simulink subsystem "RRR_rigid_joints_"  (R2021b)
settings: Solver=VariableStepAuto  StartTime=0.0  StopTime=10.0  RelTol=1e-3
undefined symbols (not defined in the file): q0, qd0
settings Model: Creator=fabioscap  LastModifiedBy=fabioscap

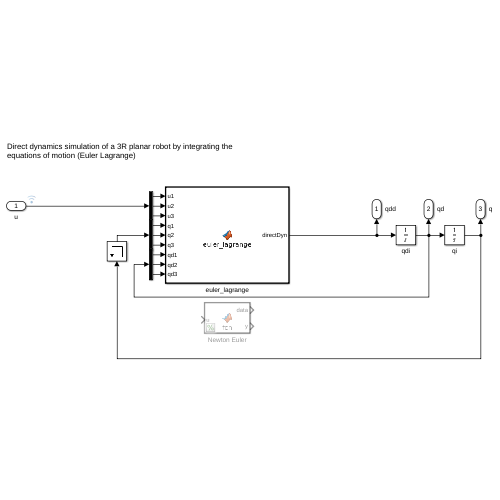
[thumbnail: Simulink's stored preview of the top-level diagram]
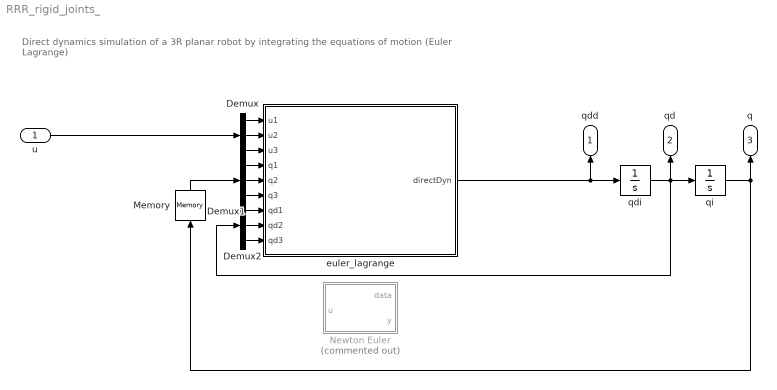
== system RRR_rigid_joints_ ==
  note: Direct dynamics simulation of a 3R planar robot by integrating the equations of motion (Euler Lagrange)
  u : Inport  PortDimensions=3
  Demux : Demux  Outputs=3
  Demux1 : Demux  Outputs=3
  Demux2 : Demux  Outputs=3
  Memory : Memory
  Newton Euler : MATLAB Function  Commented=on  TreatAsAtomicUnit=on
  euler_lagrange : MATLAB Function  TreatAsAtomicUnit=on
  qdi : Integrator  InitialCondition=qd0
  qi : Integrator  InitialCondition=q0
  qdd : Outport
  qd : Outport  Port=2
  q : Outport  Port=3  PortDimensions=3
  wires:
  Demux/2 -> euler_lagrange/2(u2)
  u/1 -> Demux/1
  Demux2/3 -> euler_lagrange/9(qd3)
  Demux/3 -> euler_lagrange/3(u3)
  euler_lagrange/1(directDyn) -> qdi/1, qdd/1
  Demux1/3 -> euler_lagrange/6(q3)
  Demux1/2 -> euler_lagrange/5(q2)
  qi/1 -> Memory/1, q/1
  Demux2/2 -> euler_lagrange/8(qd2)
  Memory/1 -> Demux1/1
  Demux2/1 -> euler_lagrange/7(qd1)
  qdi/1 -> Demux2/1, qi/1, qd/1
  Demux1/1 -> euler_lagrange/4(q1)
  Demux/1 -> euler_lagrange/1(u1)

== matlab function RRR_rigid_joints_/euler_lagrange ==
  data: u1 input; directDyn output; u2 input; u3 input; q1 input; q2 input; q3 input; qd1 input; qd2 input; qd3 input
function directDyn = euler_lagrange(u1,u2,u3,q1,q2,q3,qd1,qd2,qd3)
%#codegen

%    This function was generated by the Symbolic Math Toolbox version 9.0.
%    22-Jul-2022 17:48:26

t2 = cos(q2);
t3 = cos(q3);
t4 = sin(q2);
t5 = sin(q3);
t6 = q2+q3;
t7 = qd1.^2;
t8 = qd2.^2;
t9 = qd3.^2;
t16 = u1.*8.0;
t10 = t2.^2;
t11 = t3.^2;
t12 = t5.^2;
t13 = t5.^3;
t14 = cos(t6);
t15 = sin(t6);
t20 = t2.*u1.*1.2e+1;
t21 = t2.*u2.*1.2e+1;
t22 = t2.*u3.*1.2e+1;
t25 = qd1.*qd2.*t4.*2.4e+1;
t26 = qd1.*qd3.*t5.*3.2e+1;
t27 = qd2.*qd3.*t5.*3.2e+1;
t33 = t4.*t8.*1.2e+1;
t34 = t5.*t9.*1.6e+1;
t41 = t2.*t3.*u3.*1.8e+1;
t54 = t2.*t5.*t7.*6.0;
t55 = t2.*t5.*t8.*6.0;
t56 = t2.*t5.*t9.*6.0;
t60 = qd1.*qd2.*t2.*t5.*1.2e+1;
t61 = qd1.*qd3.*t2.*t5.*1.2e+1;
t62 = qd2.*qd3.*t2.*t5.*1.2e+1;
t63 = qd1.*qd2.*t2.*t4.*3.6e+1;
t73 = t2.*t4.*t7.*1.8e+1;
t74 = t2.*t4.*t8.*1.8e+1;
t91 = qd1.*qd2.*t2.*t3.*t5.*1.8e+1;
t110 = t2.*t3.*t5.*t7.*9.0;
t111 = t2.*t3.*t5.*t8.*9.0;
t17 = t14.^2;
t18 = t15.^2;
t19 = t15.^3;
t23 = t11.*u1.*6.0;
t24 = t11.*u2.*6.0;
t28 = t10.*9.0;
t29 = t11.*1.2e+1;
t30 = t12.*4.8e+1;
t31 = -t21;
t35 = t12.*u1.*2.4e+1;
t36 = t12.*u2.*2.4e+1;
t37 = -t26;
t38 = -t27;
t40 = t14.*u3.*1.2e+1;
t43 = -t34;
t45 = t3.*t14.*u1.*6.0;
t46 = t3.*t14.*u2.*6.0;
t47 = t3.*t14.*u3.*6.0;
t51 = t7.*t15.*4.0;
t52 = t8.*t15.*4.0;
t53 = t9.*t15.*4.0;
t57 = qd1.*qd2.*t15.*8.0;
t58 = qd1.*qd3.*t15.*8.0;
t59 = qd2.*qd3.*t15.*8.0;
t65 = t5.*t15.*u1.*2.4e+1;
t66 = t5.*t15.*u2.*2.4e+1;
t67 = t5.*t15.*u3.*2.4e+1;
t70 = -t54;
t71 = -t55;
t72 = -t56;
t75 = -t60;
t76 = -t61;
t77 = -t62;
t78 = qd1.*qd2.*t4.*t11.*1.8e+1;
t80 = t2.*t3.*t14.*9.0;
t81 = t2.*t7.*t15.*6.0;
t82 = t5.*t7.*t14.*6.0;
t83 = t2.*t8.*t15.*6.0;
t84 = t5.*t8.*t14.*6.0;
t85 = t2.*t9.*t15.*6.0;
t86 = qd1.*qd2.*t2.*t15.*1.2e+1;
t87 = qd1.*qd2.*t5.*t14.*1.2e+1;
t88 = qd1.*qd3.*t2.*t15.*1.2e+1;
t89 = qd2.*qd3.*t2.*t15.*1.2e+1;
t90 = t2.*t5.*t15.*3.6e+1;
t93 = qd1.*qd2.*t11.*t15.*6.0;
t94 = qd1.*qd3.*t11.*t15.*6.0;
t96 = qd2.*qd3.*t11.*t15.*6.0;
t98 = t3.*t5.*t15.*u3.*3.6e+1;
t99 = t4.*t7.*t11.*9.0;
t100 = t4.*t8.*t11.*9.0;
t101 = t4.*t7.*t12.*3.6e+1;
t102 = t4.*t8.*t12.*3.6e+1;
t103 = qd1.*qd2.*t4.*t12.*7.2e+1;
t104 = qd1.*qd2.*t3.*t5.*t14.*6.0;
t105 = qd1.*qd3.*t3.*t5.*t14.*6.0;
t106 = qd2.*qd3.*t3.*t5.*t14.*6.0;
t108 = t3.*t7.*t15.*2.4e+1;
t109 = t12.*t14.*u3.*3.6e+1;
t113 = -t91;
t114 = t7.*t11.*t15.*3.0;
t115 = t8.*t11.*t15.*3.0;
t116 = t9.*t11.*t15.*3.0;
t120 = qd1.*qd2.*t13.*t14.*3.6e+1;
t121 = t7.*t14.*t15.*6.0;
t122 = t3.*t5.*t7.*t14.*3.0;
t123 = t3.*t5.*t8.*t14.*3.0;
t124 = t3.*t5.*t9.*t14.*3.0;
t128 = qd1.*qd2.*t3.*t4.*t14.*1.8e+1;
t133 = -t110;
t134 = -t111;
t137 = t7.*t13.*t14.*1.8e+1;
t139 = t8.*t13.*t14.*1.8e+1;
t141 = qd1.*qd2.*t3.*t14.*t15.*6.0;
t142 = qd1.*qd3.*t3.*t14.*t15.*6.0;
t143 = qd2.*qd3.*t3.*t14.*t15.*6.0;
t147 = t3.*t4.*t7.*t14.*9.0;
t148 = t2.*t3.*t7.*t15.*9.0;
t149 = t3.*t4.*t8.*t14.*9.0;
t150 = t4.*t5.*t7.*t15.*3.6e+1;
t151 = t4.*t5.*t8.*t15.*3.6e+1;
t152 = qd1.*qd2.*t4.*t5.*t15.*7.2e+1;
t153 = qd1.*qd2.*t3.*t12.*t15.*3.6e+1;
t156 = t3.*t7.*t14.*t15.*3.0;
t157 = t3.*t8.*t14.*t15.*3.0;
t158 = t3.*t9.*t14.*t15.*3.0;
t159 = t3.*t5.*t14.*t15.*1.8e+1;
t163 = t2.*t7.*t14.*t15.*9.0;
t165 = t3.*t7.*t12.*t15.*1.8e+1;
t167 = t3.*t8.*t12.*t15.*1.8e+1;
t169 = qd1.*qd2.*t12.*t14.*t15.*3.6e+1;
t174 = t7.*t12.*t14.*t15.*1.8e+1;
t176 = t8.*t12.*t14.*t15.*1.8e+1;
t32 = -t24;
t39 = t17.*3.0;
t42 = -t28;
t44 = -t36;
t48 = t18.*1.2e+1;
t49 = -t40;
t50 = t17.*u2.*6.0;
t64 = -t46;
t69 = t18.*u2.*2.4e+1;
t79 = -t66;
t95 = qd1.*qd3.*t5.*t17.*6.0;
t97 = qd2.*qd3.*t5.*t17.*6.0;
t107 = -t80;
t112 = -t90;
t125 = -t104;
t126 = -t105;
t127 = -t106;
t129 = t12.*t17.*9.0;
t130 = t11.*t18.*9.0;
t131 = -t108;
t132 = -t109;
t135 = t5.*t9.*t17.*-3.0;
t136 = t4.*t7.*t17.*9.0;
t138 = t3.*t7.*t19.*1.8e+1;
t140 = t4.*t7.*t18.*3.6e+1;
t144 = -t122;
t145 = -t123;
t146 = -t124;
t154 = qd1.*qd2.*t3.*t5.*t18.*3.6e+1;
t160 = -t148;
t161 = -t153;
t164 = -t159;
t166 = t3.*t5.*t7.*t18.*1.8e+1;
t168 = t3.*t5.*t8.*t18.*1.8e+1;
t170 = -t165;
t172 = -t167;
t175 = t5.*t7.*t14.*t18.*1.8e+1;
t68 = -t50;
t92 = -t69;
t117 = t5.*t9.*t39;
t118 = -t95;
t119 = -t97;
t155 = -t138;
t162 = -t154;
t171 = -t166;
t173 = -t168;
t177 = t29+t30+t39+t42+t48+t107+t112+t129+t130+t164+1.6e+1;
t178 = 1.0./t177;
et1 = t16+t20+t22+t23+t25+t32+t33+t35+t37+t38+t41+t43+t44+t45+t47+t49+t51+t52+t53+t57+t58+t59+t63+t65+t67+t68+t70+t71+t72+t74+t75+t76+t77+t78+t81+t82+t83+t84+t85+t86+t87+t88+t89+t92+t93+t94+t96+t98+t99+t100+t101+t102+t103+t113+t114+t115+t116+t118+t119+t120+t121+t125+t126+t127+t128+t131+t132+t133+t134+t135+t136+t137+t139+t140+t141+t142+t143+t144+t145+t146+t149+t151+t152+t155+t156+t157+t158+t160+t161+t162+t163+t169+t170+t172+t173+t175+t176-u2.*4.0e+1+u3.*3.2e+1+t4.*t7.*6.0e+1-t5.*t7.*1.6e+1-t5.*t8.*1.6e+1-t2.*u2.*2.4e+1+t3.*u3.*4.8e+1+t17.*u3.*6.0+t18.*u3.*2.4e+1-qd1.*qd2.*t5.*3.2e+1+t2.*t4.*t7.*3.6e+1-t3.*t5.*t7.*2.4e+1-t3.*t5.*t8.*2.4e+1-t5.*t7.*t17.*3.0-t5.*t8.*t17.*3.0-t2.*t14.*u3.*1.8e+1-t3.*t14.*u2.*1.2e+1;
et2 = t5.*t15.*u2.*-4.8e+1+t3.*t18.*u3.*3.6e+1-qd1.*qd2.*t3.*t5.*4.8e+1-qd1.*qd2.*t5.*t17.*6.0+t2.*t5.*t7.*t14.*9.0+t3.*t4.*t7.*t14.*1.8e+1+t2.*t5.*t8.*t14.*9.0+t4.*t5.*t7.*t15.*7.2e+1-t3.*t5.*t7.*t18.*3.6e+1+t7.*t12.*t14.*t15.*3.6e+1-t5.*t14.*t15.*u3.*3.6e+1+qd1.*qd2.*t2.*t5.*t14.*1.8e+1;
et3 = t20+t31+t37+t38+t43+t45+t63+t64+t65+t68+t73+t74+t79+t81+t83+t85+t86+t88+t89+t92+t118+t119-t121+t128+t131+t135+t136+t140+t141+t142+t143+t147+t148+t149+t150+t151+t152+t155+t156+t157+t158+t162+t163+t169+t171+t173+t174+t175+t176-u2.*3.2e+1+u3.*6.4e+1+t4.*t7.*4.8e+1-t5.*t7.*3.2e+1-t5.*t8.*3.2e+1-t7.*t13.*4.8e+1-t8.*t13.*4.8e+1-t7.*t15.*1.6e+1-t7.*t19.*1.2e+1-t3.*u2.*4.8e+1+t3.*u3.*9.6e+1-t10.*u3.*1.8e+1+t11.*u3.*9.6e+1+t12.*u3.*9.6e+1-t14.*u1.*1.2e+1+t14.*u2.*1.2e+1+t17.*u3.*3.0e+1+t18.*u3.*4.8e+1-qd1.*qd2.*t5.*6.4e+1-qd1.*qd2.*t13.*9.6e+1+t3.*t4.*t7.*7.2e+1-t3.*t5.*t7.*4.8e+1-t3.*t5.*t8.*4.8e+1-t3.*t5.*t9.*2.4e+1;
et4 = t5.*t7.*t11.*-4.8e+1-t5.*t8.*t11.*4.8e+1-t4.*t7.*t14.*1.8e+1-t4.*t8.*t14.*1.8e+1-t5.*t7.*t17.*1.5e+1-t5.*t7.*t18.*1.2e+1-t5.*t8.*t17.*1.5e+1-t5.*t8.*t18.*1.2e+1-t7.*t11.*t15.*4.8e+1-t7.*t12.*t15.*4.8e+1-t7.*t11.*t19.*3.6e+1-t7.*t13.*t17.*3.6e+1-t8.*t14.*t15.*6.0-t8.*t13.*t17.*3.6e+1-t9.*t14.*t15.*6.0-t7.*t15.*t17.*1.2e+1+t5.*t7.*t28+t5.*t8.*t28+t7.*t15.*t28+t2.*t3.*u1.*1.8e+1-t2.*t3.*u2.*1.8e+1+t2.*t14.*u2.*1.8e+1-t2.*t14.*u3.*3.6e+1-t3.*t18.*u2.*3.6e+1+t3.*t18.*u3.*7.2e+1-t12.*t14.*u1.*3.6e+1+t12.*t14.*u2.*3.6e+1+t11.*t18.*u3.*7.2e+1+t12.*t17.*u3.*7.2e+1-qd1.*qd2.*t3.*t5.*9.6e+1;
et5 = qd1.*qd3.*t3.*t5.*-4.8e+1-qd2.*qd3.*t3.*t5.*4.8e+1+qd1.*qd2.*t5.*t10.*1.8e+1-qd1.*qd2.*t5.*t11.*9.6e+1-qd1.*qd2.*t4.*t14.*3.6e+1-qd1.*qd2.*t5.*t17.*3.0e+1-qd1.*qd2.*t5.*t18.*2.4e+1-qd1.*qd2.*t14.*t15.*1.2e+1-qd1.*qd2.*t13.*t17.*7.2e+1-qd1.*qd3.*t14.*t15.*1.2e+1-qd2.*qd3.*t14.*t15.*1.2e+1+t2.*t3.*t4.*t7.*2.7e+1+t2.*t3.*t4.*t8.*2.7e+1-t2.*t4.*t7.*t14.*2.7e+1+t2.*t3.*t8.*t15.*9.0+t2.*t5.*t7.*t14.*1.8e+1+t2.*t3.*t9.*t15.*9.0+t2.*t5.*t8.*t14.*1.8e+1+t2.*t5.*t9.*t14.*9.0+t2.*t5.*t7.*t18.*3.6e+1+t3.*t4.*t7.*t18.*5.4e+1+t2.*t7.*t12.*t15.*3.6e+1+t2.*t8.*t12.*t15.*3.6e+1-t4.*t7.*t12.*t14.*5.4e+1-t4.*t8.*t12.*t14.*5.4e+1-t5.*t7.*t11.*t18.*3.6e+1;
et6 = t5.*t8.*t11.*t18.*-3.6e+1-t7.*t12.*t15.*t17.*3.6e+1-t2.*t3.*t14.*u3.*7.2e+1+t3.*t5.*t15.*u1.*3.6e+1-t2.*t5.*t15.*u3.*7.2e+1-t3.*t5.*t15.*u2.*3.6e+1+t5.*t14.*t15.*u2.*3.6e+1-t5.*t14.*t15.*u3.*7.2e+1+qd1.*qd2.*t2.*t3.*t4.*5.4e+1+qd1.*qd2.*t2.*t3.*t15.*1.8e+1+qd1.*qd2.*t2.*t5.*t14.*3.6e+1+qd1.*qd3.*t2.*t3.*t15.*1.8e+1+qd1.*qd3.*t2.*t5.*t14.*1.8e+1+qd2.*qd3.*t2.*t3.*t15.*1.8e+1+qd2.*qd3.*t2.*t5.*t14.*1.8e+1+qd1.*qd2.*t2.*t12.*t15.*7.2e+1-qd1.*qd2.*t4.*t12.*t14.*1.08e+2-qd1.*qd2.*t5.*t11.*t18.*7.2e+1+t2.*t3.*t5.*t7.*t14.*3.6e+1+t2.*t3.*t5.*t8.*t14.*3.6e+1+t3.*t4.*t5.*t7.*t15.*5.4e+1+t3.*t4.*t5.*t8.*t15.*5.4e+1+t2.*t3.*t7.*t14.*t15.*3.6e+1-t4.*t5.*t7.*t14.*t15.*5.4e+1;
et7 = t3.*t5.*t7.*t14.*t18.*7.2e+1+t3.*t7.*t12.*t14.*t15.*7.2e+1+t3.*t8.*t12.*t14.*t15.*7.2e+1-t3.*t5.*t14.*t15.*u3.*1.44e+2+qd1.*qd2.*t2.*t3.*t5.*t14.*7.2e+1+qd1.*qd2.*t3.*t4.*t5.*t15.*1.08e+2+qd1.*qd2.*t3.*t12.*t14.*t15.*1.44e+2;
directDyn = [t178.*(t16+t22+t23+t25+t31+t32+t33+t35+t41+t44+t47+t49+t51+t52+t53+t57+t58+t59+t64+t67+t70+t71+t72+t73+t75+t76+t77+t78+t79+t82+t84+t87+t93+t94+t96+t98+t99+t100+t101+t102+t103+t113+t114+t115+t116+t120+t121+t125+t126+t127+t132+t133+t134+t137+t139+t144+t145+t146+t147+t150+t160+t161+t170+t171+t172+t174-u2.*8.0+t4.*t7.*1.2e+1).*(3.0./2.0);t178.*(et1+et2).*(-3.0./2.0);t178.*(et3+et4+et5+et6+et7).*(3.0./2.0)];

== matlab function RRR_rigid_joints_/Newton Euler ==
  data: data output; u input; y output
function [data, y]= fcn(u)

y = u;
